simulink model "Testing_new_propeller"  (R2020b)
settings: Solver=VariableStepAuto  StartTime=0.0  StopTime=10.0  RelTol=1e-3
settings Model: Creator=Jonathan van Zyl  LastModifiedBy=Jonathan van Zyl

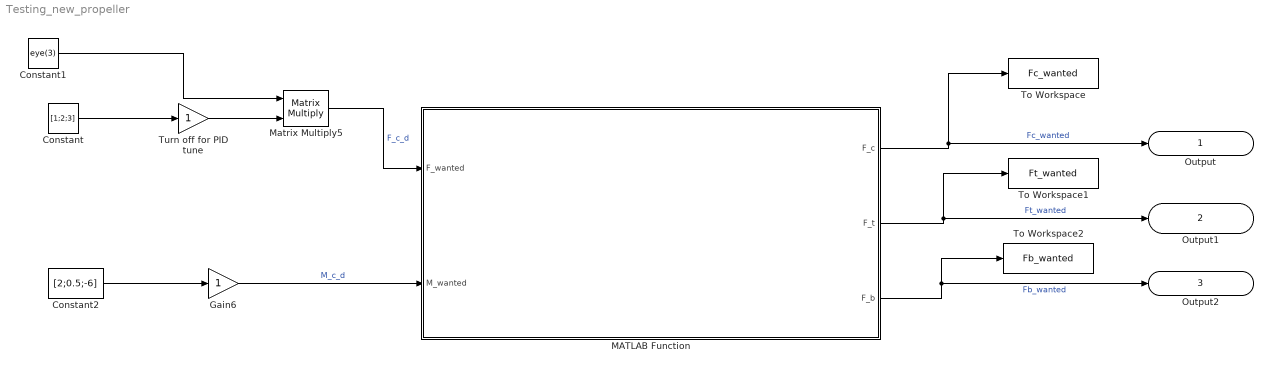
== system Testing_new_propeller ==
  Constant : Constant  Value=[1;2;3]
  Constant1 : Constant  Value=eye(3)
  Constant2 : Constant  Value=[2;0.5;-6]
  Gain6 : Gain
  MATLAB Function : MATLAB Function  TreatAsAtomicUnit=on
  Matrix Multiply5 : Product  Multiplication=Matrix(*)
  To Workspace : ToWorkspace  VariableName=Fc_wanted  SaveFormat=Timeseries  SampleTime=-1
  To Workspace1 : ToWorkspace  VariableName=Ft_wanted  SaveFormat=Timeseries  SampleTime=-1
  To Workspace2 : ToWorkspace  VariableName=Fb_wanted  SaveFormat=Timeseries  SampleTime=-1
  Turn off for PID tune : Gain
  Output : Outport
  Output1 : Outport  Port=2
  Output2 : Outport  Port=3
  wires:
  Constant2/1 -> Gain6/1
  MATLAB Function/1(F_c) -> To Workspace/1, Output/1  "Fc_wanted"
  Matrix Multiply5/1 -> MATLAB Function/1(F_wanted)  "F_c_d"
  Gain6/1 -> MATLAB Function/2(M_wanted)  "M_c_d"
  Turn off for PID tune/1 -> Matrix Multiply5/2
  MATLAB Function/3(F_b) -> Output2/1, To Workspace2/1  "Fb_wanted"
  MATLAB Function/2(F_t) -> To Workspace1/1, Output1/1  "Ft_wanted"
  Constant1/1 -> Matrix Multiply5/1
  Constant/1 -> Turn off for PID tune/1

== matlab function Testing_new_propeller/MATLAB Function ==
  data: F_wanted input; F_c output; M_wanted input; F_t output; F_b output
function [F_c, F_t, F_b] = propeller_required_forces_control(F_wanted, M_wanted)
%% New prop arms
%CATIA trans
TcgCatia = [1 0 0;
    0 -1 0;
    0 0 -1];

%Propeller arms - changed due to CATIA errors
t_1 = [1259.8002; 1300; 839.472];   %Top Front Left
t_2 = [1259.8002; -1300; 839.472];  %Top Front Right
t_3 = [-1340.1998; 1300; 839.472];  %Top Back Left
t_4 = [-1340.1998; -1300; 839.472]; %Top Back Right

b_1 = [2259.8002; 1300; -561.25];   %Bottom Front Left
b_2 = [2259.8002; -1300; -561.25];  %Bottom Front Right
b_3 = [-1340.1998; 1300; -561.25];  %Bottom Back Left
b_4 = [-1340.1998; -1300; -561.25]; %Bottom Back Right

c_1 = [-640.1998; 0; 506.566];      %Control Back Top
c_2 = [-1040.1998; 0; -493.434];    %Control Back Bottom
c_3 = [2259.8002; 0; -293.434];     %Control Front

%Propeller arms - rotated
t_1 = TcgCatia*t_1;
t1 = transpose(t_1);
t_2 = TcgCatia*t_2;
t2 = transpose(t_2);
t_3 = TcgCatia*t_3;
t3 = transpose(t_3);
t_4 = TcgCatia*t_4;
t4 = transpose(t_4);
b_1 = TcgCatia*b_1;
b1 = transpose(b_1);
b_2 = TcgCatia*b_2;
b2 = transpose(b_2);
b_3 = TcgCatia*b_3;
b3 = transpose(b_3);
b_4 = TcgCatia*b_4;
b4 = transpose(b_4);
c_1 = TcgCatia*c_1;
c1 = transpose(c_1);
c_2 = TcgCatia*c_2;
c2 = transpose(c_2);
c_3 = TcgCatia*c_3;
c3 = transpose(c_3);

prop_arms = [t1;t2;t3;t4;b1;b2;b3;b4;c1;c2;c3];

props = struct('t1', t1, 't2', t2, 't3', t3, 't4', t4, 'b1', b1, 'b2', b2, 'b3', b3, 'b4', b4, 'c1', c1, 'c2', c2, 'c3', c3);

xc_1 = props.c1(1);
yc_1 = props.c1(2);
zc_1 = props.c1(3);

xc_2 = props.c2(1);
yc_2 = props.c2(2);
zc_2 = props.c2(3);

xc_3 = props.c3(1);
yc_3 = props.c3(2);
zc_3 = props.c3(3);

xt_1 = props.t1(1);
yt_1 = props.t1(2);
zt_1 = props.t1(3);

xt_2 = props.t2(1);
yt_2 = props.t2(2);
zt_2 = props.t2(3);

xt_3 = props.t3(1);
yt_3 = props.t3(2);
zt_3 = props.t3(3);

xt_4 = props.t4(1);
yt_4 = props.t4(2);
zt_4 = props.t4(3);

xb_1 = props.b1(1);
yb_1 = props.b1(2);
zb_1 = props.b1(3);

xb_2 = props.b2(1);
yb_2 = props.b2(2);
zb_2 = props.b2(3);

xb_3 = props.b3(1);
yb_3 = props.b3(2);
zb_3 = props.b3(3);

xb_4 = props.b4(1);
yb_4 = props.b4(2);
zb_4 = props.b4(3);

%% Decompose force and moment input

F_x = F_wanted(1);
F_y = F_wanted(2);

F_z = F_wanted(3);

M_x = M_wanted(1);
M_y = M_wanted(2);
M_z = M_wanted(3);

%% Find control forces
A_control = [1 1 1;
    zc_1 -zc_2 -zc_3;
    -xc_1 -xc_2 xc_3];
A_cinv = inv(A_control);
force_control = [F_y; M_x; M_z];
controlvec = A_cinv*force_control;
F_c1 = controlvec(1);
F_c2 = controlvec(2);
F_c3 = controlvec(3);

%% Find top and bottom forces
A_tb = [-1 -1;
    2*(xt_1 + xb_1) -2*(xt_3 + xb_3)];
A_tbinv = inv(A_tb);
force_tb = [F_z; M_y];
tbvec = A_tbinv * force_tb;
f_front = tbvec(1);
F_t1 = f_front/4;
F_t2 = f_front/4;
F_b1 = f_front/4;
F_b2 = f_front/4;
f_back = tbvec(2);
F_t3 = f_back/4;
F_t4 = f_back/4;
F_b3 = f_back/4;
F_b4 = f_back/4;



%% Make matrix
F_c = [F_c1; F_c2; F_c3];
F_t = [F_t1; F_t2; F_t3; F_t4];
F_b = [F_b1; F_b2; F_b3; F_b4];
end
